simulink library "plant_cl"  (R2018b)
settings: Solver=VariableStepAuto  StartTime=0.0  StopTime=10.0  RelTol=1e-3
undefined symbols (not defined in the file or in its folder): batteryMaxEnergy, initializeBussesFromBlock
libraries: simulink x1, groundStation_cl x1, tethers_cl x1, vehicle_cl x1, winch_cl x1
settings Model: Creator=mcobb  LastModifiedBy=mcobb

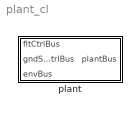
== system plant_cl ==
  plant : Subsystem  LoadFcn=initializeBussesFromBlock(gcb)  InitFcn=initializeBussesFromBlock(gcb)  StartFcn=initializeBussesFromBlock(gcb)  VariantControl=VSS_plant_modularPlant

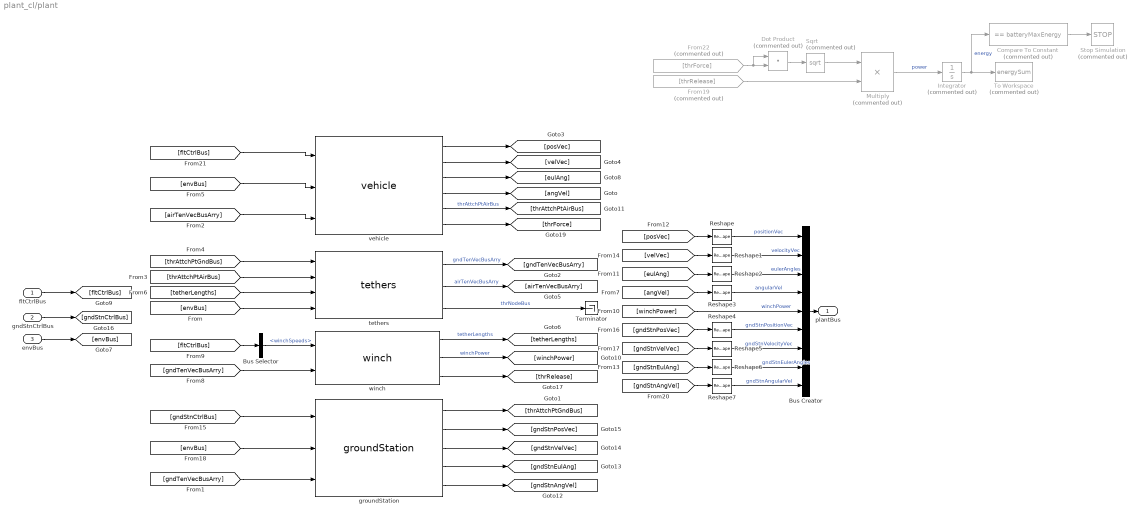
== system plant_cl/plant ==
  fltCtrlBus : Inport  OutDataTypeStr=Bus: fltCtrlBus
  gndStnCtrlBus : Inport  Port=2  OutDataTypeStr=Bus: gndStnCtrlBus
  envBus : Inport  Port=3  OutDataTypeStr=Bus: envBus
  Bus Creator : BusCreator  Inputs=9  OutDataTypeStr=Bus: plantBus
  Bus Selector : BusSelector  OutputSignals=winchSpeeds
  Compare To Constant : simulink/Logic and Bit Operations/Compare To Constant  Commented=on  relop===  const=batteryMaxEnergy  OutDataTypeStr=boolean
  Dot Product : DotProduct  Commented=on  InputSameDT=on  OutDataTypeStr=Inherit: Inherit via internal rule
  From19 : From  Commented=on  GotoTag=thrRelease
  From22 : From  Commented=on  GotoTag=thrForce
  Integrator : Integrator  Commented=on
  Multiply : Product  Commented=on
  Reshape{,1..7} (8 alike) : Reshape  OutputDimensionality=Column vector (2-D)
  Sqrt : Sqrt  Commented=on  SaturateOnIntegerOverflow=on
  Stop Simulation : Stop  Commented=on
  Terminator : Terminator
  To Workspace : ToWorkspace  Commented=on  VariableName=energySum  SaveFormat=Timeseries  SampleTime=-1
  groundStation : groundStation_cl/groundStation  SystemSampleTime=-1
  tethers : tethers_cl/tethers  SystemSampleTime=-1
  vehicle : vehicle_cl/vehicle  SystemSampleTime=-1
  winch : winch_cl/winch  SystemSampleTime=-1
  plantBus : Outport  OutDataTypeStr=Bus: plantBus
  wires:
  envBus/1 -> [envBus]
  fltCtrlBus/1 -> [fltCtrlBus]
  Bus Creator/1 -> plantBus/1
  Reshape/1 -> Bus Creator/1  "positionVec"
  Reshape2/1 -> Bus Creator/3  "eulerAngles"
  Reshape1/1 -> Bus Creator/2  "velocityVec"
  winch/1 -> [tetherLengths]  "tetherLengths"
  [posVec] -> Reshape/1
  [velVec] -> Reshape1/1
  [eulAng] -> Reshape2/1
  vehicle/3 -> [eulAng]
  vehicle/1 -> [posVec]
  vehicle/5 -> [thrAttchPtAirBus]  "thrAttchPtAirBus"
  vehicle/2 -> [velVec]
  vehicle/4 -> [angVel]
  [envBus] -> tethers/4
  groundStation/1 -> [thrAttchPtGndBus]
  tethers/1 -> [gndTenVecBusArry]  "gndTenVecBusArry"
  tethers/2 -> [airTenVecBusArry]  "airTenVecBusArry"
  tethers/3 -> Terminator/1  "thrNodeBus"
  [gndTenVecBusArry] -> groundStation/3
  [airTenVecBusArry] -> vehicle/3
  [thrAttchPtAirBus] -> tethers/2
  [thrAttchPtGndBus] -> tethers/1
  [tetherLengths] -> tethers/3
  [envBus] -> groundStation/2
  [gndStnCtrlBus] -> groundStation/1
  [fltCtrlBus] -> vehicle/1
  [envBus] -> vehicle/2
  [fltCtrlBus] -> Bus Selector/1
  [angVel] -> Reshape3/1
  Reshape3/1 -> Bus Creator/4  "angularVel"
  [gndTenVecBusArry] -> winch/2
  winch/2 -> [winchPower]  "winchPower"
  [winchPower] -> Bus Creator/5  "winchPower"
  [gndStnAngVel] -> Reshape7/1
  [gndStnEulAng] -> Reshape6/1
  [gndStnVelVec] -> Reshape5/1
  [gndStnPosVec] -> Reshape4/1
  Reshape4/1 -> Bus Creator/6  "gndStnPositionVec"
  Reshape5/1 -> Bus Creator/7  "gndStnVelocityVec"
  Reshape6/1 -> Bus Creator/8  "gndStnEulerAngles"
  Reshape7/1 -> Bus Creator/9  "gndStnAngularVel"
  groundStation/2 -> [gndStnPosVec]
  groundStation/3 -> [gndStnVelVec]
  groundStation/4 -> [gndStnEulAng]
  groundStation/5 -> [gndStnAngVel]
  gndStnCtrlBus/1 -> [gndStnCtrlBus]
  Bus Selector/1 -> winch/1  "<winchSpeeds>"
  winch/3 -> [thrRelease]
  From22/1 -> Dot Product/1, Dot Product/2
  Dot Product/1 -> Sqrt/1
  Sqrt/1 -> Multiply/1
  From19/1 -> Multiply/2
  Multiply/1 -> Integrator/1  "power"
  Integrator/1 -> Compare To Constant/1, To Workspace/1  "energy"
  vehicle/6 -> [thrForce]
  Compare To Constant/1 -> Stop Simulation/1
